simulink model "SmartStormwaterModel_CEE4800"  (R2020a)
settings: Solver=VariableStepAuto  StartTime=0.0  StopTime=10.0  RelTol=1e-3
values from neighbouring files (symbols this model uses):
  basin2 = 13890000    [data.mat]
  k = 1    [data.mat]
  n = 0.02    [data.mat]
  R = 0.75    [data.mat]
  S = 0.2    [data.mat]
libraries: simulink x10
settings Model: Creator=lydialagorga  LastModifiedBy=lydialagorga

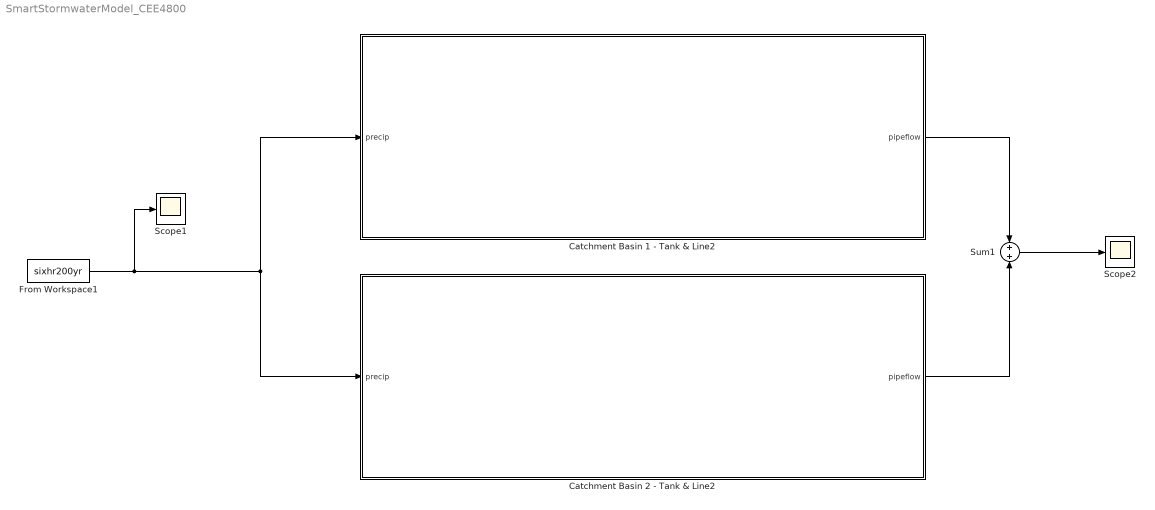
== system SmartStormwaterModel_CEE4800 ==
  Catchment Basin 1 - Tank & Line2 : Subsystem
  Catchment Basin 2 - Tank & Line2 : Subsystem
  From Workspace1 : FromWorkspace  VariableName=sixhr200yr  SampleTime=1
  Scope1 : Scope
  Scope2 : Scope
  Sum1 : Sum  Inputs=+|+
  wires:
  Sum1/1 -> Scope2/1
  From Workspace1/1 -> Scope1/1, Catchment Basin 1 - Tank & Line2/1(precip), Catchment Basin 2 - Tank & Line2/1(precip)
  Catchment Basin 1 - Tank & Line2/1(pipeflow) -> Sum1/1
  Catchment Basin 2 - Tank & Line2/1(pipeflow) -> Sum1/2

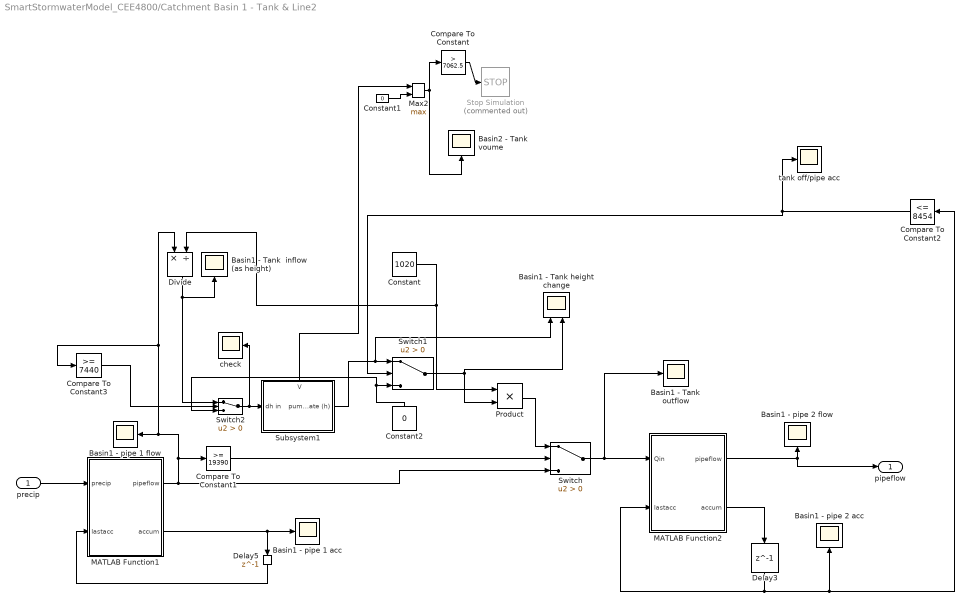
== system SmartStormwaterModel_CEE4800/Catchment Basin 1 - Tank & Line2 ==
  precip : Inport
  "  Basin1 - pipe 1 flow" : Scope
  " Basin1 - pipe 1 acc" : Scope
  " Basin2 - Tank voume" : Scope
  Basin1 - Tank  inflow (as height) : Scope
  Basin1 - Tank height change : Scope  NumInputPorts=2
  Basin1 - Tank outflow : Scope
  Basin1 - pipe 2 acc : Scope
  Basin1 - pipe 2 flow : Scope
  Compare To Constant : simulink/Logic and Bit Operations/Compare To Constant  relop=>  const=7062.5  OutDataTypeStr=boolean
  Compare To Constant1 : simulink/Logic and Bit Operations/Compare To Constant  relop=>=  const=19390  OutDataTypeStr=boolean
  Compare To Constant2 : simulink/Logic and Bit Operations/Compare To Constant  relop=<=  const=8454  OutDataTypeStr=boolean
  Compare To Constant3 : simulink/Logic and Bit Operations/Compare To Constant  relop=>=  const=7440  OutDataTypeStr=boolean
  Constant : Constant  Value=1020
  Constant1 : Constant  Value=0
  Constant2 : Constant  Value=0  SampleTime=1
  Delay3 : Delay  DelayLength=1  InitialCondition=0
  Delay5 : Delay  DelayLength=1  InitialCondition=0
  Divide : Product  Inputs=*/
  MATLAB Function1 : MATLAB Function  TreatAsAtomicUnit=on
  MATLAB Function2 : MATLAB Function  TreatAsAtomicUnit=on
  Max2 : MinMax  Function=max  Inputs=2
  Product : Product
  Stop Simulation : Stop  Commented=on
  Subsystem1 : Subsystem
      settings: PortSchema="{\"entries\":[{\"content\":{\"sides\":[{\"content\":{\"connectorIds\":[\"In1\"]},\"type\":\"ConnectorPlacement.EquallySpacedRectSide\",\"uuid\":\"49521410-f26e-428f-a0f4-6065ef8c5de4\"},{\"content\":{\"connectorIds\":[\"Out1\"],\"side\":\"RIGHT\"},\"type\":\"ConnectorPlacement.EquallySpacedRectSide\",\"uuid\":\"23e51712-c361-47eb-a12a-34fba58dacf0\"},{\"content\":{\"connectorIds\":[\"Out2\"],\"side\":\"TOP\"},\"type\":\"ConnectorPlacement.EquallySpacedRectSide\",\"uuid\":\"3d891762-d113-46ae-9add-fc9d38759335\"},{\"content\":{\"connectorIds\":[],\"side\":\"BOTTOM\"},\"type\":\"ConnectorPlacement.EquallySpacedRectSide\",\"uuid\":\"478163d5-2f8e-48b3-a9ce-7bd7e130e649\"}]},\"type\":\"ConnectorPlacement.EquallySpacedConnector\",\"uuid\":\"d8b883b0-28bd-4a78-a85b-3cb93156455b\"}],\"packageUris\":[\"http://schema.mathworks.com/mf0/Connector/19700101\"],\"version\":\"1.0\"}"
  Switch : Switch  Criteria=u2 > Threshold
  Switch1 : Switch  Criteria=u2 > Threshold
  Switch2 : Switch  Criteria=u2 > Threshold
  check : Scope
  tank off/pipe acc : Scope
  pipeflow : Outport
  wires:
  MATLAB Function2/1(pipeflow) -> pipeflow/1, Basin1 - pipe 2 flow/1
  Compare To Constant/1 -> Stop Simulation/1
  precip/1 -> MATLAB Function1/1(precip)
  MATLAB Function2/2(accum) -> Delay3/1
  Product/1 -> Switch/1
  Constant/1 -> Product/1, Divide/2
  Switch1/1 -> Basin1 - Tank height change/2, Product/2
  Compare To Constant2/1 -> tank off/pipe acc/1, Switch1/2
  Divide/1 -> Switch2/1, Basin1 - Tank  inflow (as height)/1
  Constant2/1 -> Switch1/3, Switch2/3
  Delay3/1 -> MATLAB Function2/2(lastacc), Basin1 - pipe 2 acc/1, Compare To Constant2/1
  MATLAB Function1/1(pipeflow) -> Compare To Constant1/1, Compare To Constant3/1, Divide/1, "  Basin1 - pipe 1 flow"/1, Switch/3
  MATLAB Function1/2(accum) -> Delay5/1, " Basin1 - pipe 1 acc"/1
  Delay5/1 -> MATLAB Function1/2(lastacc)
  Constant1/1 -> Max2/2
  Subsystem1/2(V) -> Max2/1
  Max2/1 -> Compare To Constant/1, " Basin2 - Tank voume"/1
  Compare To Constant1/1 -> Switch/2
  Switch/1 -> MATLAB Function2/1(Qin), Basin1 - Tank outflow/1
  Subsystem1/1(pump rate (h)) -> Basin1 - Tank height change/1, Switch1/1
  Switch2/1 -> check/1, Subsystem1/1(dh in)
  Compare To Constant3/1 -> Switch2/2

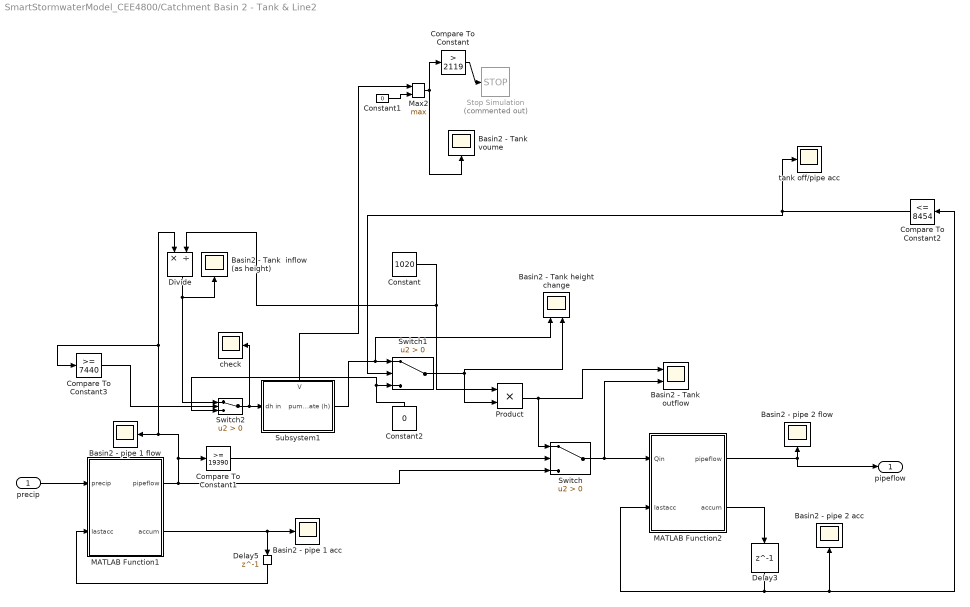
== system SmartStormwaterModel_CEE4800/Catchment Basin 2 - Tank & Line2 ==
  precip : Inport
  "  Basin2 - pipe 1 flow" : Scope
  " Basin2 - Tank voume" : Scope
  " Basin2 - pipe 1 acc" : Scope
  Basin2 - Tank  inflow (as height) : Scope
  Basin2 - Tank height change : Scope  NumInputPorts=2
  Basin2 - Tank outflow : Scope  NumInputPorts=2
  Basin2 - pipe 2 acc : Scope
  Basin2 - pipe 2 flow : Scope
  Compare To Constant : simulink/Logic and Bit Operations/Compare To Constant  relop=>  const=2119  OutDataTypeStr=boolean
  Compare To Constant1 : simulink/Logic and Bit Operations/Compare To Constant  relop=>=  const=19390  OutDataTypeStr=boolean
  Compare To Constant2 : simulink/Logic and Bit Operations/Compare To Constant  relop=<=  const=8454  OutDataTypeStr=boolean
  Compare To Constant3 : simulink/Logic and Bit Operations/Compare To Constant  relop=>=  const=7440  OutDataTypeStr=boolean
  Constant : Constant  Value=1020
  Constant1 : Constant  Value=0
  Constant2 : Constant  Value=0  SampleTime=1
  Delay3 : Delay  DelayLength=1  InitialCondition=0
  Delay5 : Delay  DelayLength=1  InitialCondition=0
  Divide : Product  Inputs=*/
  MATLAB Function1 : MATLAB Function  TreatAsAtomicUnit=on
  MATLAB Function2 : MATLAB Function  TreatAsAtomicUnit=on
  Max2 : MinMax  Function=max  Inputs=2
  Product : Product
  Stop Simulation : Stop  Commented=on
  Subsystem1 : Subsystem
      settings: PortSchema="{\"entries\":[{\"content\":{\"sides\":[{\"content\":{\"connectorIds\":[\"In1\"]},\"type\":\"ConnectorPlacement.EquallySpacedRectSide\",\"uuid\":\"49521410-f26e-428f-a0f4-6065ef8c5de4\"},{\"content\":{\"connectorIds\":[\"Out1\"],\"side\":\"RIGHT\"},\"type\":\"ConnectorPlacement.EquallySpacedRectSide\",\"uuid\":\"23e51712-c361-47eb-a12a-34fba58dacf0\"},{\"content\":{\"connectorIds\":[\"Out2\"],\"side\":\"TOP\"},\"type\":\"ConnectorPlacement.EquallySpacedRectSide\",\"uuid\":\"3d891762-d113-46ae-9add-fc9d38759335\"},{\"content\":{\"connectorIds\":[],\"side\":\"BOTTOM\"},\"type\":\"ConnectorPlacement.EquallySpacedRectSide\",\"uuid\":\"478163d5-2f8e-48b3-a9ce-7bd7e130e649\"}]},\"type\":\"ConnectorPlacement.EquallySpacedConnector\",\"uuid\":\"d8b883b0-28bd-4a78-a85b-3cb93156455b\"}],\"packageUris\":[\"http://schema.mathworks.com/mf0/Connector/19700101\"],\"version\":\"1.0\"}"
  Switch : Switch  Criteria=u2 > Threshold
  Switch1 : Switch  Criteria=u2 > Threshold
  Switch2 : Switch  Criteria=u2 > Threshold
  check : Scope
  tank off/pipe acc : Scope
  pipeflow : Outport
  wires:
  MATLAB Function2/1(pipeflow) -> pipeflow/1, Basin2 - pipe 2 flow/1
  Compare To Constant/1 -> Stop Simulation/1
  precip/1 -> MATLAB Function1/1(precip)
  MATLAB Function2/2(accum) -> Delay3/1
  Constant/1 -> Product/1, Divide/2
  Switch1/1 -> Basin2 - Tank height change/2, Product/2
  Compare To Constant2/1 -> tank off/pipe acc/1, Switch1/2
  Divide/1 -> Switch2/1, Basin2 - Tank  inflow (as height)/1
  Constant2/1 -> Switch1/3, Switch2/3
  Delay3/1 -> MATLAB Function2/2(lastacc), Basin2 - pipe 2 acc/1, Compare To Constant2/1
  MATLAB Function1/1(pipeflow) -> Compare To Constant1/1, Compare To Constant3/1, Divide/1, "  Basin2 - pipe 1 flow"/1, Switch/3
  MATLAB Function1/2(accum) -> Delay5/1, " Basin2 - pipe 1 acc"/1
  Delay5/1 -> MATLAB Function1/2(lastacc)
  Constant1/1 -> Max2/2
  Subsystem1/2(V) -> Max2/1
  Max2/1 -> Compare To Constant/1, " Basin2 - Tank voume"/1
  Compare To Constant1/1 -> Switch/2
  Switch/1 -> MATLAB Function2/1(Qin), Basin2 - Tank outflow/2
  Subsystem1/1(pump rate (h)) -> Basin2 - Tank height change/1, Switch1/1
  Switch2/1 -> check/1, Subsystem1/1(dh in)
  Compare To Constant3/1 -> Switch2/2
  Product/1 -> Switch/1, Basin2 - Tank outflow/1

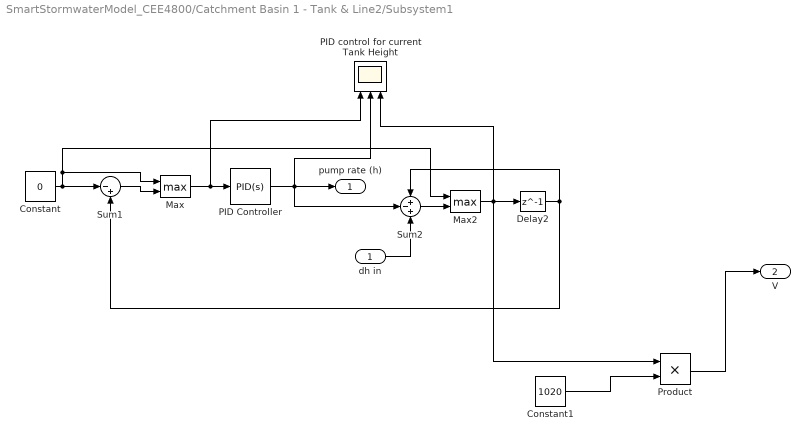
== system SmartStormwaterModel_CEE4800/Catchment Basin 1 - Tank & Line2/Subsystem1 ==
  dh in : Inport
  Constant : Constant  Value=0  SampleTime=1
  Constant1 : Constant  Value=1020
  Delay2 : Delay  DelayLength=1  InitialCondition=0
  Max : MinMax  Function=max  Inputs=2
  Max2 : MinMax  Function=max  Inputs=2
  PID Controller : simulink/Continuous/PID Controller  Controller=PID  Form=Ideal  TimeDomain=Continuous-time  UseExternalTs=off  SampleTime=1  IntegratorMethod=Forward Euler  FilterMethod=Forward Euler  ControllerParametersSource=internal  P=.9  I=.75  D=.2  UseFilter=on  N=50  TunerSelectOption=Transfer Function Based (PID Tuner App)  InitialConditionSource=internal  InitialConditionForIntegrator=0  InitialConditionForFilter=0  DifferentiatorICPrevScaledInput=0  ExternalReset=none  TrackingMode=off  Kt=1  LimitOutput=on  UpperSaturationLimit=inf  LowerSaturationLimit=0  LinearizeAsGain=on  AntiWindupMode=none  Kb=1  POutMin=0  POutMax=[]  IOutMin=[]  IOutMax=[]  DOutMin=[]  DOutMax=[]  NOutMin=[]  NOutMax=[]  SumOutMin=[]  SumOutMax=[]  SaturationOutMin=[]  SaturationOutMax=[]  PParamMin=[]  PParamMax=[]  IParamMin=[]  IParamMax=[]  DParamMin=[]  DParamMax=[]  NParamMin=[]  NParamMax=[]  KbParamMin=[]  KbParamMax=[]  KtParamMin=[]  KtParamMax=[]  KbOutMin=[]  KbOutMax=[]  KtOutMin=[]  KtOutMax=[]  IntegratorOutMin=[]  IntegratorOutMax=[]  FilterOutMin=[]  FilterOutMax=[]  SumI1OutMin=[]  SumI1OutMax=[]  SumI2OutMin=[]  SumI2OutMax=[]  SumI3OutMin=[]  SumI3OutMax=[]  SumI4OutMin=[]  SumI4OutMax=[]  SumDOutMin=[]  SumDOutMax=[]  DifferentiatorOutMin=[]  DifferentiatorOutMax=[]  FilterDiffOutCoefMin=[]  FilterDiffOutCoefMax=[]  ReciprocalOutMin=[]  ReciprocalOutMax=[]  SumDenOutMin=[]  SumDenOutMax=[]  SumNumOutMin=[]  SumNumOutMax=[]  DivideOutMin=[]  DivideOutMax=[]  UdiffTsProdOutMin=[]  UdiffTsProdOutMax=[]  NTsProdOutMin=[]  NTsProdOutMax=[]  UintegralTsProdOutMin=[]  UintegralTsProdOutMax=[]  UngainTsProdOutMin=[]  UngainTsProdOutMax=[]  IntegratorContinuousStateAttributes=''  IntegratorStateMustResolveToSignalObject=off  IntegratorRTWStateStorageClass=Auto  FilterContinuousStateAttributes=''  FilterStateMustResolveToSignalObject=off  FilterRTWStateStorageClass=Auto  ParallelPVariant=Passthrough  IdealPVariant=InternalParameters  IVariant=InternalParameters  DVariant=InternalParameters  IntegratorVariant=Continuous  SatVariant=Enabled  AWVariant=Passthrough  PCopyVariant=Disabled  TRVariant=Disabled  FdbkBlocksVariant=Forward  IdealPFdbkVariant=Disabled  SatFdbkVariant=Disabled  DerivativeFilterVariant=ContFilter  NVariant=InternalParameters  NCopyVariant=Disabled  FilterICVariant=InternalICsFilter  IntegratorICVariant=InternalICs  ExternalResetVariant=Disabled  TRSumVariant=Passthrough  SumFdbkVariant=Disabled  SumVariant=Sum_PID  TsampFilterVariant=InternalTs  TsampNgainVariant=Passthrough  TsampIntegralVariant=Passthrough
  PID control for current Tank Height : Scope  NumInputPorts=3
  Product : Product
  Sum1 : Sum  Inputs=|-+  OutMin=0
  Sum2 : Sum  Inputs=+-+  OutMin=0
  pump rate (h) : Outport
  V : Outport  Port=2
  wires:
  Delay2/1 -> Sum1/2, Sum2/1
  Sum1/1 -> Max/2
  Sum2/1 -> Max2/2
  Max/1 -> PID control for current Tank Height/1, PID Controller/1
  Max2/1 -> PID control for current Tank Height/3, Product/1, Delay2/1
  PID Controller/1 -> pump rate (h)/1, Sum2/2, PID control for current Tank Height/2
  dh in/1 -> Sum2/3
  Constant/1 -> Sum1/1, Max/1, Max2/1
  Product/1 -> V/1
  Constant1/1 -> Product/2

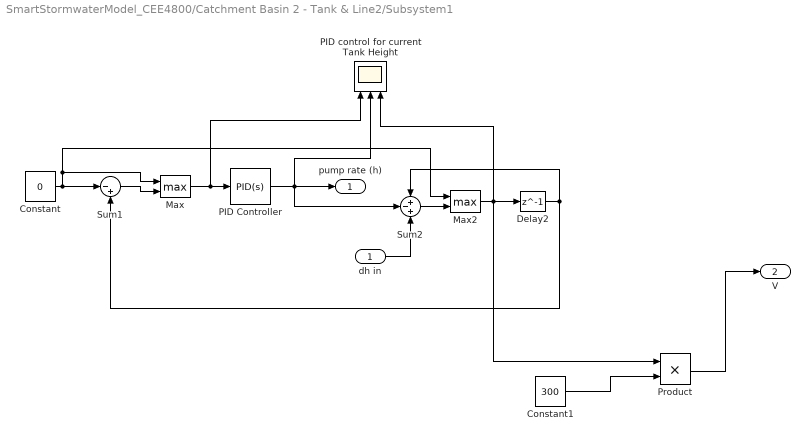
== system SmartStormwaterModel_CEE4800/Catchment Basin 2 - Tank & Line2/Subsystem1 ==
  dh in : Inport
  Constant : Constant  Value=0  SampleTime=1
  Constant1 : Constant  Value=300
  Delay2 : Delay  DelayLength=1  InitialCondition=0
  Max : MinMax  Function=max  Inputs=2
  Max2 : MinMax  Function=max  Inputs=2
  PID Controller : simulink/Continuous/PID Controller  Controller=PID  Form=Ideal  TimeDomain=Continuous-time  UseExternalTs=off  SampleTime=1  IntegratorMethod=Forward Euler  FilterMethod=Forward Euler  ControllerParametersSource=internal  P=.9  I=.75  D=.2  UseFilter=on  N=50  TunerSelectOption=Transfer Function Based (PID Tuner App)  InitialConditionSource=internal  InitialConditionForIntegrator=0  InitialConditionForFilter=0  DifferentiatorICPrevScaledInput=0  ExternalReset=none  TrackingMode=off  Kt=1  LimitOutput=on  UpperSaturationLimit=inf  LowerSaturationLimit=0  LinearizeAsGain=on  AntiWindupMode=none  Kb=1  POutMin=0  POutMax=[]  IOutMin=[]  IOutMax=[]  DOutMin=[]  DOutMax=[]  NOutMin=[]  NOutMax=[]  SumOutMin=[]  SumOutMax=[]  SaturationOutMin=[]  SaturationOutMax=[]  PParamMin=[]  PParamMax=[]  IParamMin=[]  IParamMax=[]  DParamMin=[]  DParamMax=[]  NParamMin=[]  NParamMax=[]  KbParamMin=[]  KbParamMax=[]  KtParamMin=[]  KtParamMax=[]  KbOutMin=[]  KbOutMax=[]  KtOutMin=[]  KtOutMax=[]  IntegratorOutMin=[]  IntegratorOutMax=[]  FilterOutMin=[]  FilterOutMax=[]  SumI1OutMin=[]  SumI1OutMax=[]  SumI2OutMin=[]  SumI2OutMax=[]  SumI3OutMin=[]  SumI3OutMax=[]  SumI4OutMin=[]  SumI4OutMax=[]  SumDOutMin=[]  SumDOutMax=[]  DifferentiatorOutMin=[]  DifferentiatorOutMax=[]  FilterDiffOutCoefMin=[]  FilterDiffOutCoefMax=[]  ReciprocalOutMin=[]  ReciprocalOutMax=[]  SumDenOutMin=[]  SumDenOutMax=[]  SumNumOutMin=[]  SumNumOutMax=[]  DivideOutMin=[]  DivideOutMax=[]  UdiffTsProdOutMin=[]  UdiffTsProdOutMax=[]  NTsProdOutMin=[]  NTsProdOutMax=[]  UintegralTsProdOutMin=[]  UintegralTsProdOutMax=[]  UngainTsProdOutMin=[]  UngainTsProdOutMax=[]  IntegratorContinuousStateAttributes=''  IntegratorStateMustResolveToSignalObject=off  IntegratorRTWStateStorageClass=Auto  FilterContinuousStateAttributes=''  FilterStateMustResolveToSignalObject=off  FilterRTWStateStorageClass=Auto  ParallelPVariant=Passthrough  IdealPVariant=InternalParameters  IVariant=InternalParameters  DVariant=InternalParameters  IntegratorVariant=Continuous  SatVariant=Enabled  AWVariant=Passthrough  PCopyVariant=Disabled  TRVariant=Disabled  FdbkBlocksVariant=Forward  IdealPFdbkVariant=Disabled  SatFdbkVariant=Disabled  DerivativeFilterVariant=ContFilter  NVariant=InternalParameters  NCopyVariant=Disabled  FilterICVariant=InternalICsFilter  IntegratorICVariant=InternalICs  ExternalResetVariant=Disabled  TRSumVariant=Passthrough  SumFdbkVariant=Disabled  SumVariant=Sum_PID  TsampFilterVariant=InternalTs  TsampNgainVariant=Passthrough  TsampIntegralVariant=Passthrough
  PID control for current Tank Height : Scope  NumInputPorts=3
  Product : Product
  Sum1 : Sum  Inputs=|-+  OutMin=0
  Sum2 : Sum  Inputs=+-+  OutMin=0
  pump rate (h) : Outport
  V : Outport  Port=2
  wires:
  Delay2/1 -> Sum1/2, Sum2/1
  Sum1/1 -> Max/2
  Sum2/1 -> Max2/2
  Max/1 -> PID control for current Tank Height/1, PID Controller/1
  Max2/1 -> PID control for current Tank Height/3, Product/1, Delay2/1
  PID Controller/1 -> pump rate (h)/1, Sum2/2, PID control for current Tank Height/2
  dh in/1 -> Sum2/3
  Constant/1 -> Sum1/1, Max/1, Max2/1
  Product/1 -> V/1
  Constant1/1 -> Product/2

== matlab function SmartStormwaterModel_CEE4800/Catchment Basin 2 - Tank & Line2/MATLAB Function1 ==
  data: pipeflow output; precip input; k parameter; n parameter; R parameter; S parameter; basin2 parameter; accum output; lastacc input
function [pipeflow, accum]  = pipeflow(precip, k, n, R, S, basin2,lastacc)
% v = k*n*R^0.63*S^.54
% cross sectional area: pi*r^2
% v = velocity; n = roughness; R = hydraulic radius; S = slope; k =
% conversions
pipeflowMax=7440;
pipeflow = precip*basin2*0.5635;
% v = k*n*R^0.63*S^.54; %should be 
% Ax = pi*R^2;
% pipeflowMax = v*Ax; %pipe flow out is 4.82 m3/s
% if water coming in is below max, it flows in normally
% if above max, then it flows according to the max flow
accum = 0;
if pipeflow > pipeflowMax
    if pipeflow >= 19390
    pipeflowMax = 19390;
    end
tempPipeflow = pipeflowMax;
accum = lastacc + pipeflow - tempPipeflow;
    while accum < 0
      tempPipeflow=tempPipeflow-1;
      accum = lastacc + pipeflow - tempPipeflow;
    end
    pipeflow=tempPipeflow;
end
end
% h = precip*clock; %calculates the accumulated precipitation
% Qout = C*sqrt(h); 
% dPdt = pipeflow - Qout; %change in volume; 
% % where if dVdt > volume of tank, there's a back up in system
% 
% % dPdt = basin1*precip + wateracc - pipeflow; %water remaining to be assimilated

== matlab function SmartStormwaterModel_CEE4800/Catchment Basin 2 - Tank & Line2/MATLAB Function2 ==
  data: pipeflow output; Qin input; accum output; lastacc input
function [pipeflow, accum]  = pipeflow(Qin, lastacc)
% v = k*n*R^0.63*S^.54
% cross sectional area: pi*r^2
% v = velocity; n = roughness; R = hydraulic radius; S = slope; k =
% conversions
pipeflowMax=7440;
pipeflow = Qin;
% v = k*n*R^0.63*S^.54; %should be 
% Ax = pi*R^2;
% pipeflowMax = v*Ax; %pipe flow out is 4.82 m3/s
% if water coming in is below max, it flows in normally
% if above max, then it flows according to the max flow
accum = 0;
if pipeflow > pipeflowMax
    if pipeflow >= 19390
    pipeflowMax = 19390;
    end
tempPipeflow = pipeflowMax;
accum = lastacc + pipeflow - tempPipeflow;
    while accum < 0
      tempPipeflow=tempPipeflow-1;
      accum = lastacc + pipeflow - tempPipeflow;
    end
    pipeflow=tempPipeflow;
end
end
% h = precip*clock; %calculates the accumulated precipitation
% Qout = C*sqrt(h); 
% dPdt = pipeflow - Qout; %change in volume; 
% % where if dVdt > volume of tank, there's a back up in system
% 
% % dPdt = basin1*precip + wateracc - pipeflow; %water remaining to be assimilated

== matlab function SmartStormwaterModel_CEE4800/Catchment Basin 1 - Tank & Line2/MATLAB Function1 ==
  data: pipeflow output; precip input; k parameter; n parameter; R parameter; S parameter; basin2 parameter; accum output; lastacc input
function [pipeflow, accum]  = pipeflow(precip, k, n, R, S, basin2,lastacc)
% v = k*n*R^0.63*S^.54
% cross sectional area: pi*r^2
% v = velocity; n = roughness; R = hydraulic radius; S = slope; k =
% conversions
pipeflowMax=7440;
pipeflow = precip*basin2*0.5635;
% v = k*n*R^0.63*S^.54; %should be 
% Ax = pi*R^2;
% pipeflowMax = v*Ax; %pipe flow out is 4.82 m3/s
% if water coming in is below max, it flows in normally
% if above max, then it flows according to the max flow
accum = 0;
if pipeflow > pipeflowMax
    if pipeflow >= 19390
    pipeflowMax = 19390;
    end
tempPipeflow = pipeflowMax;
accum = lastacc + pipeflow - tempPipeflow;
    while accum < 0
      tempPipeflow=tempPipeflow-1;
      accum = lastacc + pipeflow - tempPipeflow;
    end
    pipeflow=tempPipeflow;
end
end
% h = precip*clock; %calculates the accumulated precipitation
% Qout = C*sqrt(h); 
% dPdt = pipeflow - Qout; %change in volume; 
% % where if dVdt > volume of tank, there's a back up in system
% 
% % dPdt = basin1*precip + wateracc - pipeflow; %water remaining to be assimilated

== matlab function SmartStormwaterModel_CEE4800/Catchment Basin 1 - Tank & Line2/MATLAB Function2 ==
  data: pipeflow output; Qin input; accum output; lastacc input
function [pipeflow, accum]  = pipeflow(Qin, lastacc)
% v = k*n*R^0.63*S^.54
% cross sectional area: pi*r^2
% v = velocity; n = roughness; R = hydraulic radius; S = slope; k =
% conversions
pipeflowMax=7440;
pipeflow = Qin;
% v = k*n*R^0.63*S^.54; %should be 
% Ax = pi*R^2;
% pipeflowMax = v*Ax; %pipe flow out is 4.82 m3/s
% if water coming in is below max, it flows in normally
% if above max, then it flows according to the max flow
accum = 0;
if pipeflow > pipeflowMax
    if pipeflow >= 19390
    pipeflowMax = 19390;
    end
tempPipeflow = pipeflowMax;
accum = lastacc + pipeflow - tempPipeflow;
    while accum < 0
      tempPipeflow=tempPipeflow-1;
      accum = lastacc + pipeflow - tempPipeflow;
    end
    pipeflow=tempPipeflow;
end
end
% h = precip*clock; %calculates the accumulated precipitation
% Qout = C*sqrt(h); 
% dPdt = pipeflow - Qout; %change in volume; 
% % where if dVdt > volume of tank, there's a back up in system
% 
% % dPdt = basin1*precip + wateracc - pipeflow; %water remaining to be assimilated
